simulink subsystem "PLL"  (R2022b)
settings: Solver=VariableStepAuto  StartTime=0.0  StopTime=10.0  RelTol=1e-3
libraries: msbPllFoundation x1
settings Model: Creator=Ali-Laptop  LastModifiedBy=Ali-Laptop

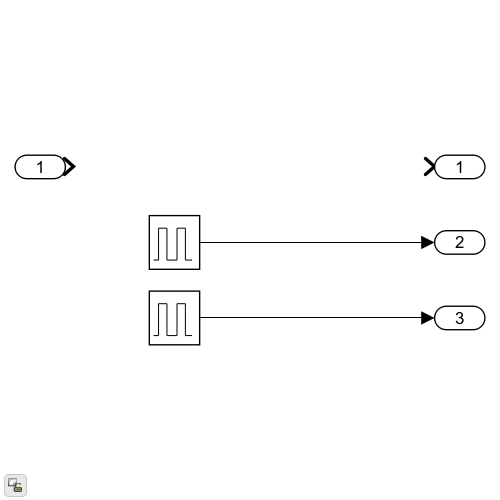
[thumbnail: Simulink's stored preview of the top-level diagram]
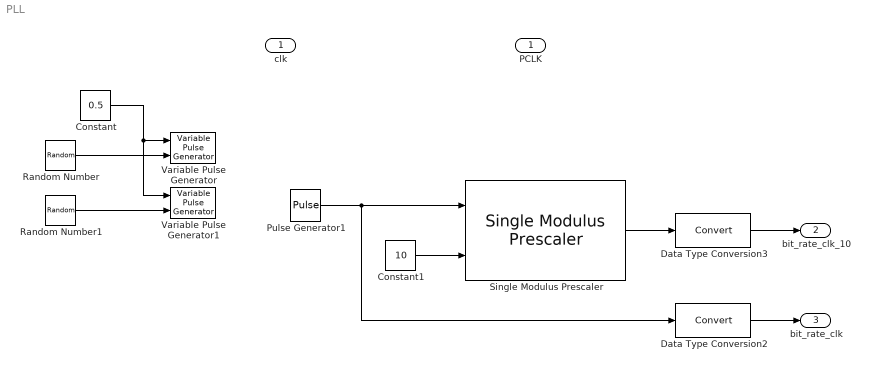
== system PLL ==
  clk : Inport
  Constant : Constant  Value=0.5  SampleTime=-1
  Constant1 : Constant  Value=10
  Data Type Conversion2 : DataTypeConversion  SaturateOnIntegerOverflow=off  RndMeth=Floor
  Data Type Conversion3 : DataTypeConversion  SaturateOnIntegerOverflow=off  RndMeth=Floor
  Pulse Generator1 : DiscretePulseGenerator  PulseType=Time based  Period=2.0002e-10  PulseWidth=50
  Random Number : RandomNumber  Mean=2e-9  Variance=0  SampleTime=1
  Random Number1 : RandomNumber  Mean=2e-10  Variance=0  SampleTime=1
  Single Modulus Prescaler : msbPllFoundation/Single Modulus Prescaler  ExtraBuffer=off  NBuffer=1
  Variable Pulse Generator : VariablePulseGenerator  SampleTime=0.1
  Variable Pulse Generator1 : VariablePulseGenerator  SampleTime=0.1
  PCLK : Outport
  bit_rate_clk_10 : Outport  Port=2
  bit_rate_clk : Outport  Port=3
  wires:
  Pulse Generator1/1 -> Data Type Conversion2/1, Single Modulus Prescaler/1
  Constant/1 -> Variable Pulse Generator/1, Variable Pulse Generator1/1
  Random Number/1 -> Variable Pulse Generator/2
  Random Number1/1 -> Variable Pulse Generator1/2
  Constant1/1 -> Single Modulus Prescaler/2
  Data Type Conversion2/1 -> bit_rate_clk/1
  Single Modulus Prescaler/1 -> Data Type Conversion3/1
  Data Type Conversion3/1 -> bit_rate_clk_10/1
